simulink model "inclass0910"  (R2022b)
settings: Solver=VariableStepAuto  StartTime=0.0  StopTime=20.0  RelTol=1e-3
settings Model: Creator=sprinkle  LastModifiedBy=sprinkle

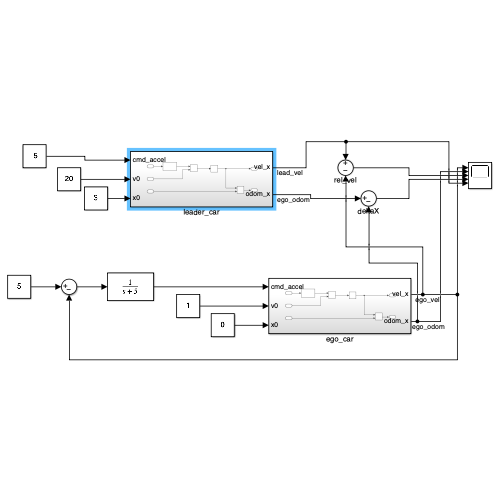
[thumbnail: Simulink's stored preview of the top-level diagram]
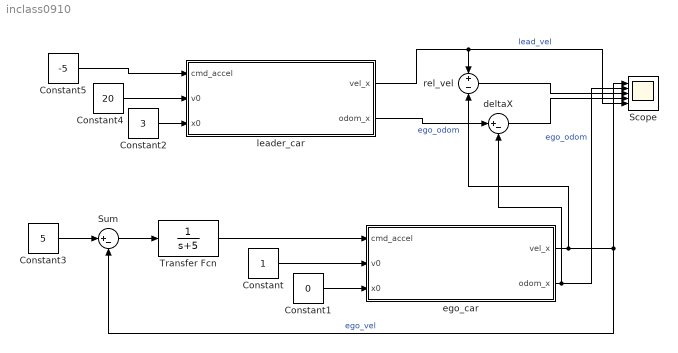
== system inclass0910 ==
  Constant : Constant
  Constant1 : Constant  Value=0
  Constant2 : Constant  Value=3
  Constant3 : Constant  Value=5
  Constant4 : Constant  Value=20
  Constant5 : Constant  Value=-5
  Scope : Scope  NumInputPorts=5
  Sum : Sum  Inputs=|+-
  Transfer Fcn : TransferFcn  Denominator=[1 5]
  deltaX : Sum  Inputs=|+-
  ego_car : Subsystem
  leader_car : Subsystem
  rel_vel : Sum  Inputs=+-
  wires:
  Constant/1 -> ego_car/2(v0)
  Constant1/1 -> ego_car/3(x0)
  Transfer Fcn/1 -> ego_car/1(cmd_accel)
  ego_car/1(vel_x) -> rel_vel/2, Sum/2, Scope/1  "ego_vel"
  ego_car/2(odom_x) -> Scope/2, deltaX/2  "ego_odom"
  Sum/1 -> Transfer Fcn/1
  Constant3/1 -> Sum/1
  Constant2/1 -> leader_car/3(x0)
  Constant4/1 -> leader_car/2(v0)
  Constant5/1 -> leader_car/1(cmd_accel)
  leader_car/1(vel_x) -> Scope/5, rel_vel/1  "lead_vel"
  rel_vel/1 -> Scope/3
  leader_car/2(odom_x) -> deltaX/1  "ego_odom"
  deltaX/1 -> Scope/4

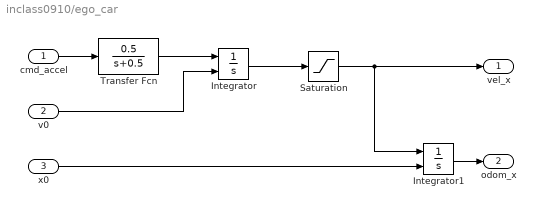
== system inclass0910/ego_car ==
  cmd_accel : Inport
  v0 : Inport  Port=2
  x0 : Inport  Port=3
  Integrator : Integrator  InitialConditionSource=external
  Integrator1 : Integrator  InitialConditionSource=external
  Saturation : Saturate  UpperLimit=80  LowerLimit=0
  Transfer Fcn : TransferFcn  Numerator=[0.5]  Denominator=[1 0.5]
  vel_x : Outport
  odom_x : Outport  Port=2
  wires:
  v0/1 -> Integrator/2
  cmd_accel/1 -> Transfer Fcn/1
  Transfer Fcn/1 -> Integrator/1
  Integrator1/1 -> odom_x/1
  Integrator/1 -> Saturation/1
  x0/1 -> Integrator1/2
  Saturation/1 -> vel_x/1, Integrator1/1

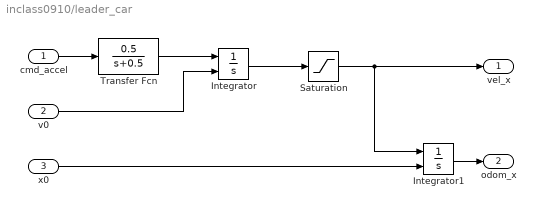
== system inclass0910/leader_car ==
  cmd_accel : Inport
  v0 : Inport  Port=2
  x0 : Inport  Port=3
  Integrator : Integrator  InitialConditionSource=external
  Integrator1 : Integrator  InitialConditionSource=external
  Saturation : Saturate  UpperLimit=80  LowerLimit=0
  Transfer Fcn : TransferFcn  Numerator=[0.5]  Denominator=[1 0.5]
  vel_x : Outport
  odom_x : Outport  Port=2
  wires:
  v0/1 -> Integrator/2
  cmd_accel/1 -> Transfer Fcn/1
  Transfer Fcn/1 -> Integrator/1
  Integrator1/1 -> odom_x/1
  Integrator/1 -> Saturation/1
  x0/1 -> Integrator1/2
  Saturation/1 -> vel_x/1, Integrator1/1
